simulink model "drone_model"  (R2020b)
settings: Solver=ode45  StartTime=0.0  StopTime=50  MaxStep=0.005  RelTol=1e-3
libraries: sharedtransform x3, pid_lib x3, shared6dof x1, uavutilslib x1, aerolibutil x1
settings Model: Creator=tesla  LastModifiedBy=tesla

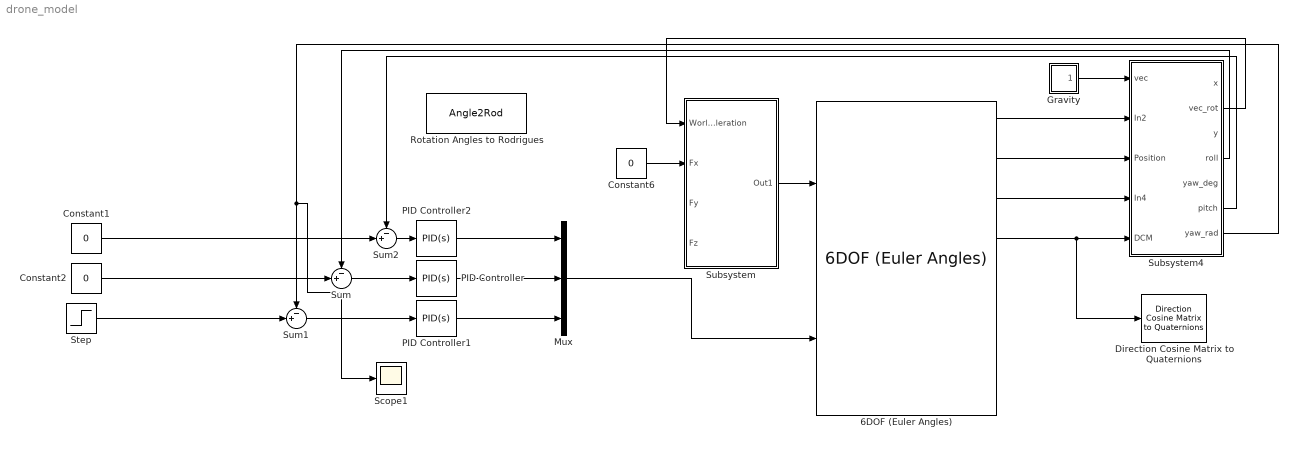
== system drone_model ==
  6DOF (Euler Angles) : shared6dof/6DOF (Euler Angles)  units=Metric (MKS)  mtype=Fixed  rep=Euler Angles  xme_0=[0 0 0]  Vm_0=[0 0 0]  eul_0=[0 0 0]  pm_0=[0 0 0]  mass_0=1.0  mass_e=0.5  mass_f=2.0  inertia=eye(3)*5  inertia_e=eye(3)  inertia_f=2*eye(3)  k_quat=1.0  vre_flag=on  abi_flag=off  aMode=0  xme_statename=''  Vm_statename=''  eul_statename=''  quat_statename=''  pm_statename=''  mass_statename=''
      settings: SourceProductBaseCode=AE,PW,MT,UV,VE,VP
  Constant1 : Constant  Value=0
  Constant2 : Constant  Value=0
  Constant6 : Constant  Value=0
  Direction Cosine Matrix to Quaternions : sharedtransform/Direction Cosine Matrix  to Quaternions  aMode=0  action=None  tolerance=eps(2)
      settings: SourceProductBaseCode=AE,PW,MT,UV,VE,VP
  Gravity : Subsystem
  Mux : Mux  Inputs=3
  PID Controller : pid_lib/PID Controller  Controller=PID  Form=Parallel  TimeDomain=Continuous-time  UseExternalTs=off  SampleTime=-1  IntegratorMethod=Forward Euler  FilterMethod=Forward Euler  ControllerParametersSource=internal  P=12  I=3  D=7.5  UseFilter=on  N=100  TunerSelectOption=Transfer Function Based (PID Tuner App)  InitialConditionSource=internal  InitialConditionForIntegrator=0  InitialConditionForFilter=0  DifferentiatorICPrevScaledInput=0  ExternalReset=none  TrackingMode=off  Kt=1  LimitOutput=on  SatLimitsSource=internal  UpperSaturationLimit=0.5  LowerSaturationLimit=-0.5  LinearizeAsGain=on  AntiWindupMode=clamping  Kb=1  POutMin=[]  POutMax=[]  IOutMin=[]  IOutMax=[]  DOutMin=[]  DOutMax=[]  NOutMin=[]  NOutMax=[]  SumOutMin=[]  SumOutMax=[]  SaturationOutMin=[]  SaturationOutMax=[]  PParamMin=[]  PParamMax=[]  IParamMin=[]  IParamMax=[]  DParamMin=[]  DParamMax=[]  NParamMin=[]  NParamMax=[]  KbParamMin=[]  KbParamMax=[]  KtParamMin=[]  KtParamMax=[]  KbOutMin=[]  KbOutMax=[]  KtOutMin=[]  KtOutMax=[]  IntegratorOutMin=[]  IntegratorOutMax=[]  FilterOutMin=[]  FilterOutMax=[]  SumI1OutMin=[]  SumI1OutMax=[]  SumI2OutMin=[]  SumI2OutMax=[]  SumI3OutMin=[]  SumI3OutMax=[]  SumI4OutMin=[]  SumI4OutMax=[]  SumDOutMin=[]  SumDOutMax=[]  DifferentiatorOutMin=[]  DifferentiatorOutMax=[]  FilterDiffOutCoefMin=[]  FilterDiffOutCoefMax=[]  ReciprocalOutMin=[]  ReciprocalOutMax=[]  SumDenOutMin=[]  SumDenOutMax=[]  SumNumOutMin=[]  SumNumOutMax=[]  DivideOutMin=[]  DivideOutMax=[]  UdiffTsProdOutMin=[]  UdiffTsProdOutMax=[]  NTsProdOutMin=[]  NTsProdOutMax=[]  UintegralTsProdOutMin=[]  UintegralTsProdOutMax=[]  UngainTsProdOutMin=[]  UngainTsProdOutMax=[]  IntegratorContinuousStateAttributes=''  IntegratorStateMustResolveToSignalObject=off  IntegratorRTWStateStorageClass=Auto  FilterContinuousStateAttributes=''  FilterStateMustResolveToSignalObject=off  FilterRTWStateStorageClass=Auto  ParallelPVariant=InternalParameters  IdealPVariant=Disabled  IVariant=InternalParameters  DVariant=InternalParameters  IntegratorVariant=Continuous  SatVariant=Enabled  AWVariant=ContClampingParallel  PCopyVariant=Disabled  TRVariant=Disabled  FdbkBlocksVariant=Forward  IdealPFdbkVariant=Disabled  SatFdbkVariant=Disabled  DerivativeFilterVariant=ContFilter  NVariant=InternalParameters  NCopyVariant=Disabled  FilterICVariant=InternalICsFilter  IntegratorICVariant=InternalICs  ExternalResetVariant=Disabled  TRSumVariant=Passthrough  SumFdbkVariant=Disabled  SumVariant=Sum_PID  TsampFilterVariant=InternalTs  TsampNgainVariant=Passthrough  TsampIntegralVariant=Passthrough  ExternalSaturationOutDataTypeStr=Inherit: Same as second input
  PID Controller1 : pid_lib/PID Controller  Controller=PID  Form=Parallel  TimeDomain=Continuous-time  UseExternalTs=off  SampleTime=-1  IntegratorMethod=Forward Euler  FilterMethod=Forward Euler  ControllerParametersSource=internal  P=12  I=3  D=10  UseFilter=on  N=25  TunerSelectOption=Transfer Function Based (PID Tuner App)  InitialConditionSource=internal  InitialConditionForIntegrator=0  InitialConditionForFilter=0  DifferentiatorICPrevScaledInput=0  ExternalReset=none  TrackingMode=off  Kt=1  LimitOutput=on  SatLimitsSource=internal  UpperSaturationLimit=0.5  LowerSaturationLimit=-0.5  LinearizeAsGain=on  AntiWindupMode=clamping  Kb=1  POutMin=[]  POutMax=[]  IOutMin=[]  IOutMax=[]  DOutMin=[]  DOutMax=[]  NOutMin=[]  NOutMax=[]  SumOutMin=[]  SumOutMax=[]  SaturationOutMin=[]  SaturationOutMax=[]  PParamMin=[]  PParamMax=[]  IParamMin=[]  IParamMax=[]  DParamMin=[]  DParamMax=[]  NParamMin=[]  NParamMax=[]  KbParamMin=[]  KbParamMax=[]  KtParamMin=[]  KtParamMax=[]  KbOutMin=[]  KbOutMax=[]  KtOutMin=[]  KtOutMax=[]  IntegratorOutMin=[]  IntegratorOutMax=[]  FilterOutMin=[]  FilterOutMax=[]  SumI1OutMin=[]  SumI1OutMax=[]  SumI2OutMin=[]  SumI2OutMax=[]  SumI3OutMin=[]  SumI3OutMax=[]  SumI4OutMin=[]  SumI4OutMax=[]  SumDOutMin=[]  SumDOutMax=[]  DifferentiatorOutMin=[]  DifferentiatorOutMax=[]  FilterDiffOutCoefMin=[]  FilterDiffOutCoefMax=[]  ReciprocalOutMin=[]  ReciprocalOutMax=[]  SumDenOutMin=[]  SumDenOutMax=[]  SumNumOutMin=[]  SumNumOutMax=[]  DivideOutMin=[]  DivideOutMax=[]  UdiffTsProdOutMin=[]  UdiffTsProdOutMax=[]  NTsProdOutMin=[]  NTsProdOutMax=[]  UintegralTsProdOutMin=[]  UintegralTsProdOutMax=[]  UngainTsProdOutMin=[]  UngainTsProdOutMax=[]  IntegratorContinuousStateAttributes=''  IntegratorStateMustResolveToSignalObject=off  IntegratorRTWStateStorageClass=Auto  FilterContinuousStateAttributes=''  FilterStateMustResolveToSignalObject=off  FilterRTWStateStorageClass=Auto  ParallelPVariant=InternalParameters  IdealPVariant=Disabled  IVariant=InternalParameters  DVariant=InternalParameters  IntegratorVariant=Continuous  SatVariant=Enabled  AWVariant=ContClampingParallel  PCopyVariant=Disabled  TRVariant=Disabled  FdbkBlocksVariant=Forward  IdealPFdbkVariant=Disabled  SatFdbkVariant=Disabled  DerivativeFilterVariant=ContFilter  NVariant=InternalParameters  NCopyVariant=Disabled  FilterICVariant=InternalICsFilter  IntegratorICVariant=InternalICs  ExternalResetVariant=Disabled  TRSumVariant=Passthrough  SumFdbkVariant=Disabled  SumVariant=Sum_PID  TsampFilterVariant=InternalTs  TsampNgainVariant=Passthrough  TsampIntegralVariant=Passthrough  ExternalSaturationOutDataTypeStr=Inherit: Same as second input
  PID Controller2 : pid_lib/PID Controller  Controller=PID  Form=Parallel  TimeDomain=Continuous-time  UseExternalTs=off  SampleTime=-1  IntegratorMethod=Forward Euler  FilterMethod=Forward Euler  ControllerParametersSource=internal  P=1  I=1  D=0  UseFilter=on  N=100  TunerSelectOption=Transfer Function Based (PID Tuner App)  InitialConditionSource=internal  InitialConditionForIntegrator=0  InitialConditionForFilter=0  DifferentiatorICPrevScaledInput=0  ExternalReset=none  TrackingMode=off  Kt=1  LimitOutput=on  SatLimitsSource=internal  UpperSaturationLimit=0.5  LowerSaturationLimit=-0.5  LinearizeAsGain=on  AntiWindupMode=none  Kb=1  POutMin=[]  POutMax=[]  IOutMin=[]  IOutMax=[]  DOutMin=[]  DOutMax=[]  NOutMin=[]  NOutMax=[]  SumOutMin=[]  SumOutMax=[]  SaturationOutMin=[]  SaturationOutMax=[]  PParamMin=[]  PParamMax=[]  IParamMin=[]  IParamMax=[]  DParamMin=[]  DParamMax=[]  NParamMin=[]  NParamMax=[]  KbParamMin=[]  KbParamMax=[]  KtParamMin=[]  KtParamMax=[]  KbOutMin=[]  KbOutMax=[]  KtOutMin=[]  KtOutMax=[]  IntegratorOutMin=[]  IntegratorOutMax=[]  FilterOutMin=[]  FilterOutMax=[]  SumI1OutMin=[]  SumI1OutMax=[]  SumI2OutMin=[]  SumI2OutMax=[]  SumI3OutMin=[]  SumI3OutMax=[]  SumI4OutMin=[]  SumI4OutMax=[]  SumDOutMin=[]  SumDOutMax=[]  DifferentiatorOutMin=[]  DifferentiatorOutMax=[]  FilterDiffOutCoefMin=[]  FilterDiffOutCoefMax=[]  ReciprocalOutMin=[]  ReciprocalOutMax=[]  SumDenOutMin=[]  SumDenOutMax=[]  SumNumOutMin=[]  SumNumOutMax=[]  DivideOutMin=[]  DivideOutMax=[]  UdiffTsProdOutMin=[]  UdiffTsProdOutMax=[]  NTsProdOutMin=[]  NTsProdOutMax=[]  UintegralTsProdOutMin=[]  UintegralTsProdOutMax=[]  UngainTsProdOutMin=[]  UngainTsProdOutMax=[]  IntegratorContinuousStateAttributes=''  IntegratorStateMustResolveToSignalObject=off  IntegratorRTWStateStorageClass=Auto  FilterContinuousStateAttributes=''  FilterStateMustResolveToSignalObject=off  FilterRTWStateStorageClass=Auto  ParallelPVariant=InternalParameters  IdealPVariant=Disabled  IVariant=InternalParameters  DVariant=InternalParameters  IntegratorVariant=Continuous  SatVariant=Enabled  AWVariant=Passthrough  PCopyVariant=Disabled  TRVariant=Disabled  FdbkBlocksVariant=Forward  IdealPFdbkVariant=Disabled  SatFdbkVariant=Disabled  DerivativeFilterVariant=ContFilter  NVariant=InternalParameters  NCopyVariant=Disabled  FilterICVariant=InternalICsFilter  IntegratorICVariant=InternalICs  ExternalResetVariant=Disabled  TRSumVariant=Passthrough  SumFdbkVariant=Disabled  SumVariant=Sum_PID  TsampFilterVariant=InternalTs  TsampNgainVariant=Passthrough  TsampIntegralVariant=Passthrough  ExternalSaturationOutDataTypeStr=Inherit: Same as second input
  Rotation Angles to Rodrigues : Angle2Rod
      settings: AttributesFormatString=Rotation Order: %<rotationOrder>
  Scope1 : Scope
  Step : Step  Time=15  After=0  SampleTime=0
  Subsystem : Subsystem
  Subsystem4 : Subsystem
  Sum : Sum  Inputs=-+|
  Sum1 : Sum  Inputs=-+|
  Sum2 : Sum  Inputs=-+|
  wires:
  Constant1/1 -> Sum2/2
  Sum/1 -> PID Controller/1
  Sum1/1 -> PID Controller1/1
  Step/1 -> Sum1/2
  6DOF (Euler Angles)/1 -> Subsystem4/2(In2)
  6DOF (Euler Angles)/2 -> Subsystem4/3(Position)
  6DOF (Euler Angles)/3 -> Subsystem4/4(In4)
  6DOF (Euler Angles)/4 -> Direction Cosine Matrix to Quaternions/1, Subsystem4/5(DCM)
  Sum2/1 -> PID Controller2/1
  Subsystem4/2(vec_rot) -> Subsystem/1(World Acceleration)
  Constant6/1 -> Subsystem/2(Fx)
  Subsystem/1(Out1) -> 6DOF (Euler Angles)/1
  Constant2/1 -> Sum/2
  Gravity/1(Out1) -> Subsystem4/1(vec)
  PID Controller/1 -> Mux/2
  PID Controller1/1 -> Mux/3
  PID Controller2/1 -> Mux/1
  Mux/1 -> 6DOF (Euler Angles)/2
  Subsystem4/6(pitch) -> Sum2/1
  Subsystem4/4(roll) -> Sum/1
  Subsystem4/7(yaw_rad) -> Scope1/1, Sum1/1

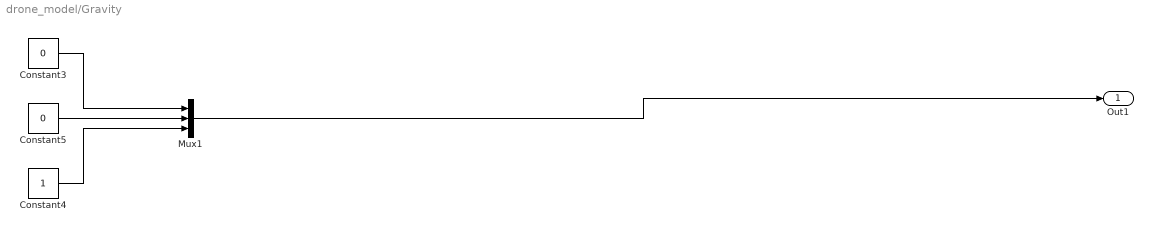
== system drone_model/Gravity ==
  Constant3 : Constant  Value=0
  Constant4 : Constant
  Constant5 : Constant  Value=0
  Mux1 : Mux  Inputs=3
  Out1 : Outport
  wires:
  Mux1/1 -> Out1/1
  Constant4/1 -> Mux1/3
  Constant5/1 -> Mux1/2
  Constant3/1 -> Mux1/1

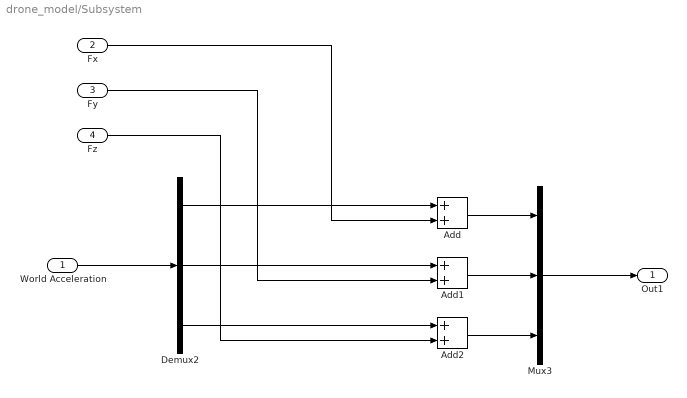
== system drone_model/Subsystem ==
  World Acceleration : Inport
  Fx : Inport  Port=2
  Fy : Inport  Port=3
  Fz : Inport  Port=4
  Add : Sum
  Add1 : Sum
  Add2 : Sum
  Demux2 : Demux  Outputs=3
  Mux3 : Mux  Inputs=3
  Out1 : Outport
  wires:
  Add/1 -> Mux3/1
  Demux2/3 -> Add2/1
  World Acceleration/1 -> Demux2/1
  Mux3/1 -> Out1/1
  Demux2/1 -> Add/1
  Fx/1 -> Add/2
  Demux2/2 -> Add1/1
  Add1/1 -> Mux3/2
  Fy/1 -> Add1/2
  Add2/1 -> Mux3/3
  Fz/1 -> Add2/2

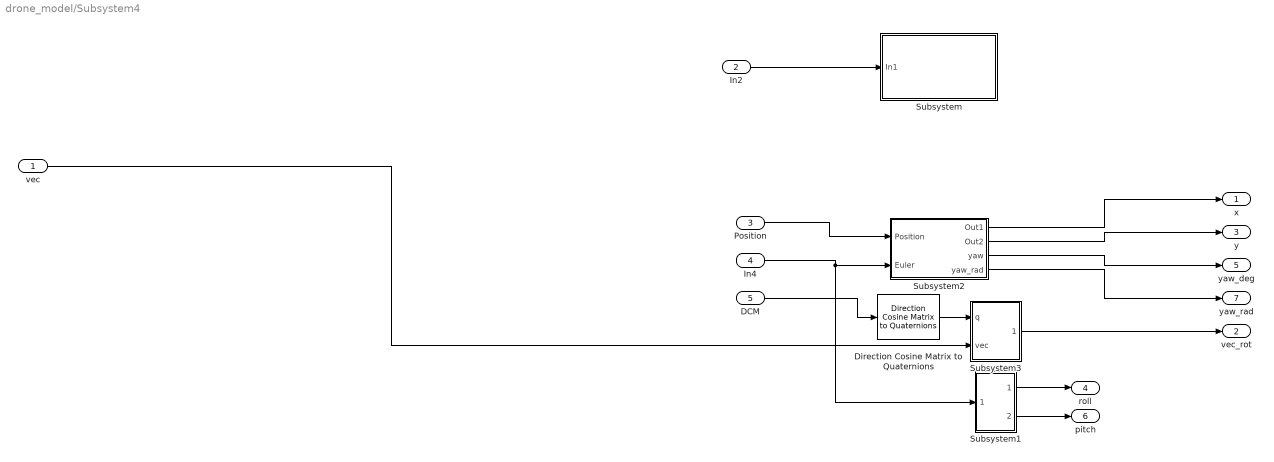
== system drone_model/Subsystem4 ==
  vec : Inport
  In2 : Inport  Port=2
  Position : Inport  Port=3
  In4 : Inport  Port=4
  DCM : Inport  Port=5
  Direction Cosine Matrix to Quaternions : sharedtransform/Direction Cosine Matrix  to Quaternions  aMode=0  action=None  tolerance=eps(2)
      settings: SourceProductBaseCode=AE,PW,MT,UV,VE,VP
  Subsystem : Subsystem
  Subsystem1 : Subsystem
  Subsystem2 : Subsystem
  Subsystem3 : Subsystem
  x : Outport
  vec_rot : Outport  Port=2
  y : Outport  Port=3
  roll : Outport  Port=4
  yaw_deg : Outport  Port=5
  pitch : Outport  Port=6
  yaw_rad : Outport  Port=7
  wires:
  Subsystem3/1(vec_rot) -> vec_rot/1
  Subsystem2/1(Out1) -> x/1
  DCM/1 -> Direction Cosine Matrix to Quaternions/1
  Subsystem2/2(Out2) -> y/1
  vec/1 -> Subsystem3/2(vec)
  Position/1 -> Subsystem2/1(Position)
  Direction Cosine Matrix to Quaternions/1 -> Subsystem3/1(q)
  Subsystem2/3(yaw) -> yaw_deg/1
  In2/1 -> Subsystem/1(In1)
  In4/1 -> Subsystem2/2(Euler), Subsystem1/1(In1)
  Subsystem1/1(roll) -> roll/1
  Subsystem1/2(pitch) -> pitch/1
  Subsystem2/4(yaw_rad) -> yaw_rad/1

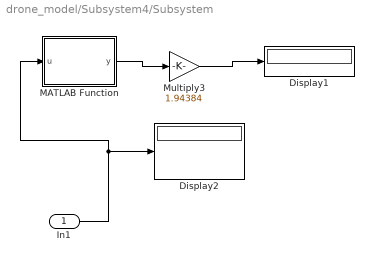
== system drone_model/Subsystem4/Subsystem ==
  In1 : Inport
  Display1 : Display
  Display2 : Display
  MATLAB Function : MATLAB Function  TreatAsAtomicUnit=on
  Multiply3 : Gain  Gain=1.94384
  wires:
  In1/1 -> MATLAB Function/1(u), Display2/1
  MATLAB Function/1(y) -> Multiply3/1
  Multiply3/1 -> Display1/1

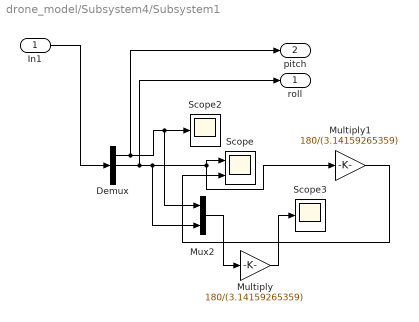
== system drone_model/Subsystem4/Subsystem1 ==
  In1 : Inport
  Demux : Demux  Outputs=3
  Multiply : Gain  Gain=180/(3.14159265359)
  Multiply1 : Gain  Gain=180/(3.14159265359)
  Mux2 : Mux  Inputs=2
  Scope : Scope  NumInputPorts=2
  Scope2 : Scope
  Scope3 : Scope
  roll : Outport
  pitch : Outport  Port=2
  wires:
  In1/1 -> Demux/1
  Mux2/1 -> Multiply/1
  Multiply1/1 -> Scope/2
  Demux/1 -> pitch/1, Mux2/1, Scope2/1
  Demux/2 -> roll/1, Mux2/2, Multiply1/1, Scope/1
  Multiply/1 -> Scope3/1

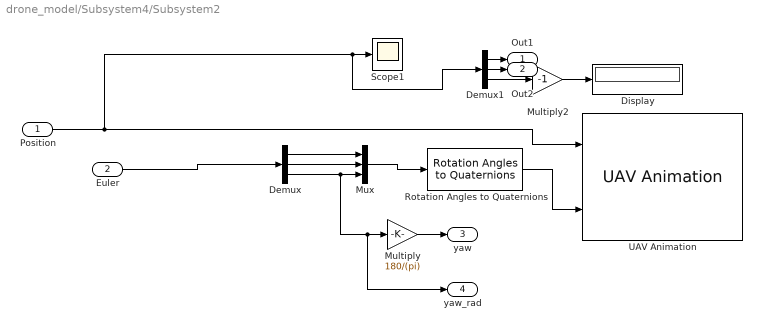
== system drone_model/Subsystem4/Subsystem2 ==
  Position : Inport
  Euler : Inport  Port=2
  Demux : Demux  Outputs=3
  Demux1 : Demux  Outputs=3
  Display : Display
  Multiply : Gain  Gain=180/(pi)
  Multiply2 : Gain  Gain=-1
  Mux : Mux  Inputs=3
  Rotation Angles to Quaternions : sharedtransform/Rotation Angles to Quaternions  rotationOrder=ZYX  aMode=aMode
      settings: SourceProductBaseCode=AE,PW,MT,UV,VE,VP
  Scope1 : Scope
  UAV Animation : uavutilslib/UAV Animation  UAVType=Multirotor  UAVSize=1  InertialZDirection=Down  SampleTime=-1
      settings: SourceProductBaseCode=UV
  Out1 : Outport
  Out2 : Outport  Port=2
  yaw : Outport  Port=3
  yaw_rad : Outport  Port=4
  wires:
  Demux1/2 -> Out2/1
  Demux1/3 -> Multiply2/1
  Demux1/1 -> Out1/1
  Euler/1 -> Demux/1
  Multiply2/1 -> Display/1
  Position/1 -> UAV Animation/1, Demux1/1, Scope1/1
  Demux/3 -> yaw_rad/1, Multiply/1, Mux/3
  Demux/1 -> Mux/1
  Demux/2 -> Mux/2
  Mux/1 -> Rotation Angles to Quaternions/1
  Multiply/1 -> yaw/1
  Rotation Angles to Quaternions/1 -> UAV Animation/2

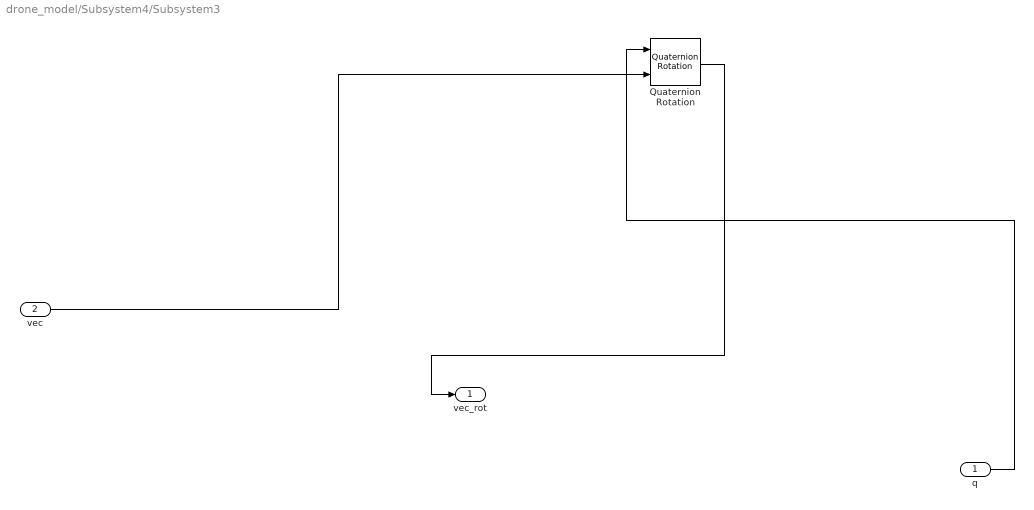
== system drone_model/Subsystem4/Subsystem3 ==
  q : Inport
  vec : Inport  Port=2
  Quaternion Rotation : aerolibutil/Quaternion Rotation
  vec_rot : Outport
  wires:
  q/1 -> Quaternion Rotation/1
  Quaternion Rotation/1 -> vec_rot/1
  vec/1 -> Quaternion Rotation/2

== matlab function drone_model/Subsystem4/Subsystem/MATLAB Function ==
  data: u input; y output
function y = fcn(u)

y = norm(u);

end
